simulink model "s0204"  (Simulink 7.0)
settings: Solver=ode45  SolverMode=SingleTasking  StartTime=0.0  StopTime=5  MaxStep=.1  RelTol=1e-3  AbsTol=1e-6
values from neighbouring files (symbols this model uses):
  T1 = 3*T1    (= 0.3)    [m0203.m]    (also in m0204.m = 0.1; m0205.m = 0.1; m0207.m = 0.1; m0221d.m = 1/a0)
  uedach = 1    [m0203.m]    (also in m0204.m = ue(i); m0207.m = ue(i))
settings Model: Creator=froriep  LastModifiedBy=froriep
settings DataIOCC: LimitDataPoints=off  SaveOutput=off  TimeSaveName=t  SignalLoggingName=sigsOut
settings OptimizationCC: BooleanDataType=off  InlineInvariantSignals=on
settings DebuggingCC: SaveWithParameterizedLinksMsg=none  SignalResolutionControl=TryResolveAllWithWarning  SolverPrmCheckMsg=none  MultiTaskDSMMsg=warning  MultiTaskCondExecSysMsg=none  StrictBusMsg=None
settings HardwareCC: TargetUnknown=on
settings RTWCC: IncludeERTFirstTime=on
settings GRTTargetCC: TargetFcnLib=ansi_tfl_tmw.mat  ModelReferenceCompliant=off  MatFileLogging=off

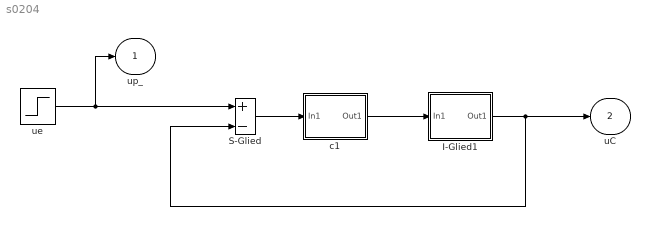
== system s0204 ==
  I-Glied1 : Subsystem  mask(I-Glied){@1=0}
      mask prompts: @1 "Anfangswert"
      mask help: I-Glied
      mask init:
      | x0=@1;
      mask Display: disp('I-Glied')
  S-Glied : Sum  Inputs=+-  OutDataType=sfix(16)  OutScaling=2^0  SaturateOnIntegerOverflow=on  InputSameDT=on
  c1 : Subsystem  mask(P-Glied){Kp=1/T1}
      mask prompts: Kp "Beiwert"
      mask help: P-Glied
      mask Display: disp('1/RC')
  ue : Step  Time=.2  After=uedach  SampleTime=0
  up_ : Outport  OutDataType=sfix(16)  OutScaling=2^0
  uC : Outport  Port=2  OutDataType=sfix(16)  OutScaling=2^0
  wires:
  ue/1 -> up_/1, S-Glied/1
  I-Glied1/1(Out1) -> uC/1, S-Glied/2
  c1/1(Out1) -> I-Glied1/1(In1)
  S-Glied/1 -> c1/1(In1)

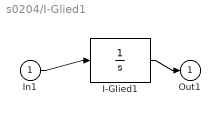
== system s0204/I-Glied1 ==
  In1 : Inport  OutDataType=sfix(16)  OutScaling=2^0
  I-Glied1 : Integrator  InitialCondition=x0
  Out1 : Outport  OutDataType=sfix(16)  OutScaling=2^0
  wires:
  In1/1 -> I-Glied1/1
  I-Glied1/1 -> Out1/1

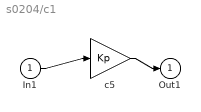
== system s0204/c1 ==
  In1 : Inport  OutDataType=sfix(16)  OutScaling=2^0
  c5 : Gain  Gain=Kp  ParameterDataType=sfix(16)  ParameterScaling=2^0  OutDataType=sfix(16)  OutScaling=2^0  SaturateOnIntegerOverflow=on
  Out1 : Outport  OutDataType=sfix(16)  OutScaling=2^0
  wires:
  c5/1 -> Out1/1
  In1/1 -> c5/1
